simulink model "Quantization"  (R2023b)
settings: Solver=VariableStepAuto  StartTime=0.0  StopTime=10.0  RelTol=1e-3
settings Model: Creator=online  LastModifiedBy=online

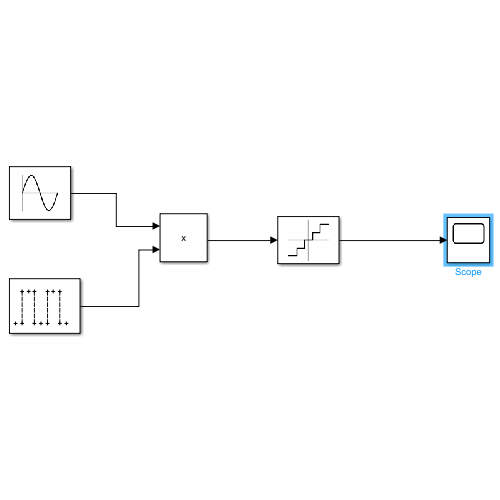
[thumbnail: Simulink's stored preview of the top-level diagram]
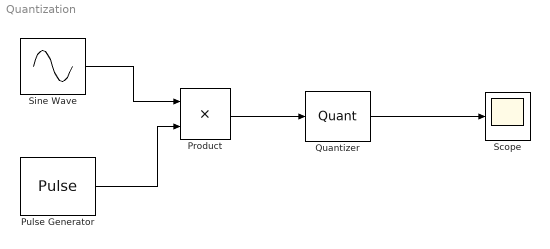
== system Quantization ==
  Product : Product
  Pulse Generator : DiscretePulseGenerator  Period=1000  PulseWidth=500  SampleTime=1/1000
  Quantizer : Quantizer  QuantizationInterval=0.25
  Scope : Scope
  Sine Wave : Sin  SampleTime=0
  wires:
  Sine Wave/1 -> Product/1
  Pulse Generator/1 -> Product/2
  Product/1 -> Quantizer/1
  Quantizer/1 -> Scope/1
